simulink model "system_id_sim"  (R2022b)
settings: Solver=FixedStepAuto  StartTime=0.0  StopTime=time_final  RelTol=1e-3  EnableMultiTasking=on
values from neighbouring files (symbols this model uses):
  input_signal_type = 3    [system_id.m]
  stepsize = 0.7    [system_id.m]
  time_final = 19    [system_id.m]
  Tss = param.encoder.Tss    [system_id.m]    (also in untitled.m)
libraries: dspsrcs4 x1
settings Model: SimulationMode=external  ExtModeTrigDuration=8  Creator=Alex Zhen  LastModifiedBy=Alex Zhen
settings OptimizationCC: DefaultUnderspecifiedDataType=single  EnhancedBackFolding=on  PassReuseOutputArgsAs=Individual arguments  MaxStackSize=1024  OptimizeBlockOrder=speed  DifferentSizesBufferReuse=on  OptimizationCustomize=off  DenormalBehavior=FlushToZero  EfficientTunableParamExpr=on
settings DebuggingCC: ParameterTunabilityLossMsg=error
settings HardwareCC: ProdBitPerChar=16  ProdBitPerInt=16  ProdBitPerPointer=32  ProdBitPerSizeT=32  ProdBitPerPtrDiffT=32  ProdLargestAtomicInteger=Integer  ProdLargestAtomicFloat=None  ProdWordSize=16  ProdLongLongMode=on  ProdHWDeviceType=Texas Instruments->C2000
settings SFSimCC: MATLABDynamicMemAlloc=off
settings RTWCC: Description=Embedded Coder  SystemTargetFile=ert.tlc  HardwareBoard=TI Delfino F28379D LaunchPad  TLCOptions=-aInlineSetEventsForThisBaseRateFcn=TLC_FALSE -aSuppressMultiTaskScheduler=TLC_FALSE -aRateBasedStepFcn=1  TemplateMakefile=ert_default_tmf  Toolchain=Texas Instruments Code Composer Studio (C2000)
settings CodeAppCC: ForceParamTrailComments=on  IgnoreCustomStorageClasses=off  OperatorAnnotations=on  SimulinkDataObjDesc=on  SFDataObjDesc=on  InsertBlockDesc=on
settings ERTTargetCC: CodeReplacementLibrary=TI C28x  SupportContinuousTime=on  ExtModeTransport=4  ExtModeStaticAlloc=on  ExtModeAutomaticAllocSize=off  ExtModeMexFile=ext_xcp  ExtModeIntrfLevel=Level2 - Open

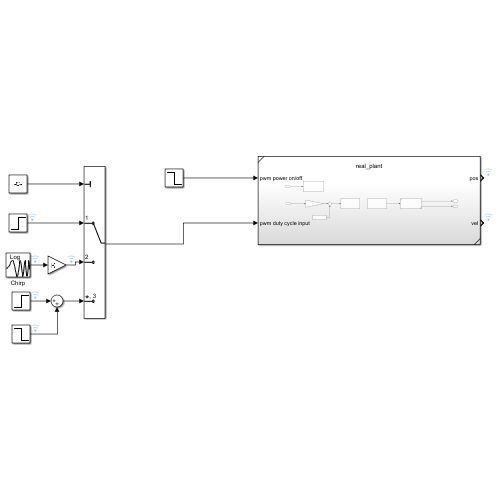
[thumbnail: Simulink's stored preview of the top-level diagram]
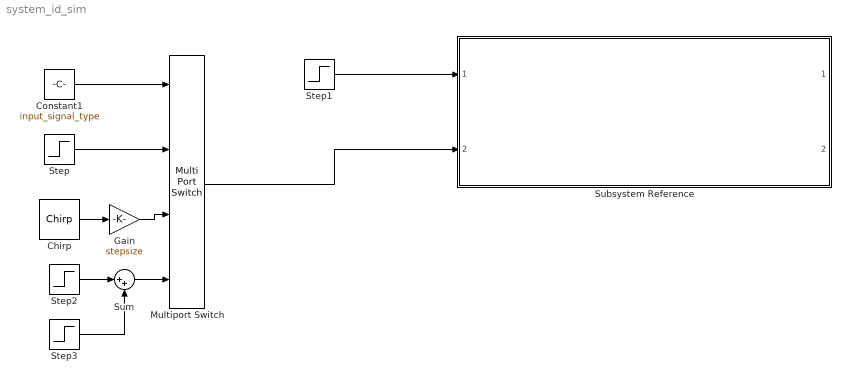
== system system_id_sim ==
  Chirp : dspsrcs4/Chirp  sweep=Logarithmic  mode=Unidirectional  f0=chirp_init_freq  f1=chirp_target_freq  t1=time_final  Tsweep=time_final  phase=0  Ts=Tss  spf=1  datatype=Double  OutputFrames=off
  Constant1 : Constant  Value=input_signal_type  SampleTime=Tss
  Gain : Gain  Gain=stepsize
  Multiport Switch : MultiPortSwitch  SaturateOnIntegerOverflow=off  InputSameDT=off
  Step : Step  Time=10  After=stepsize  SampleTime=0
  Step1 : Step  Time=time_final  Before=1  After=0  SampleTime=0
  Step2 : Step  Time=10  After=stepsize  SampleTime=0
  Step3 : Step  Time=15  After=-stepsize  SampleTime=0
  Subsystem Reference : Subsystem  ReferencedSubsystem=real_plant
  Sum : Sum  Inputs=|++
  wires:
  Step1/1 -> Subsystem Reference/1
  Step/1 -> Multiport Switch/2
  Constant1/1 -> Multiport Switch/1
  Chirp/1 -> Gain/1
  Multiport Switch/1 -> Subsystem Reference/2
  Gain/1 -> Multiport Switch/3
  Step2/1 -> Sum/1
  Step3/1 -> Sum/2
  Sum/1 -> Multiport Switch/4
